simulink model "boundedModel"  (R2019a)
settings: Solver=FixedStepAuto  StartTime=0.0  StopTime=10  FixedStep=0.001  RelTol=1e-3
settings Model: Creator=houte  LastModifiedBy=coeng

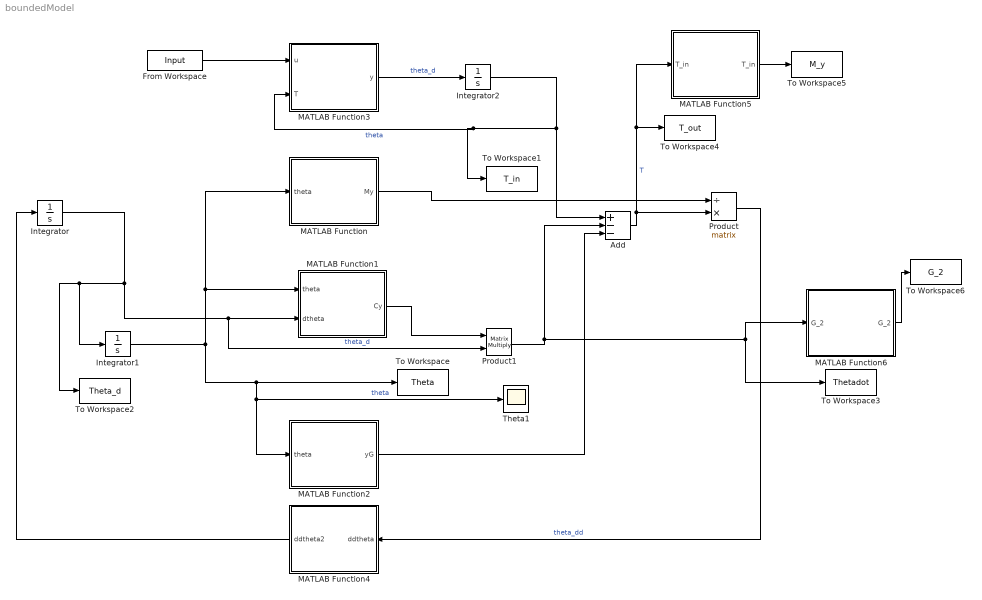
== system boundedModel ==
  Add : Sum  Inputs=+--
  From Workspace : FromWorkspace  VariableName=Input  SampleTime=0
  Integrator : Integrator  InitialCondition=[0; 0]
  Integrator1 : Integrator  InitialCondition=[0;pi]
  Integrator2 : Integrator  InitialCondition=[0;0]
  MATLAB Function : MATLAB Function  TreatAsAtomicUnit=on
  MATLAB Function1 : MATLAB Function  TreatAsAtomicUnit=on
  MATLAB Function2 : MATLAB Function  TreatAsAtomicUnit=on
  MATLAB Function3 : MATLAB Function  TreatAsAtomicUnit=on
  MATLAB Function4 : MATLAB Function  TreatAsAtomicUnit=on
  MATLAB Function5 : MATLAB Function  TreatAsAtomicUnit=on
  MATLAB Function6 : MATLAB Function  TreatAsAtomicUnit=on
  Product : Product  Inputs=/*  Multiplication=Matrix(*)
  Product1 : Product  Multiplication=Matrix(*)
  Theta1 : Scope
  To Workspace : ToWorkspace  VariableName=Theta  SaveFormat=Timeseries  SampleTime=-1
  To Workspace1 : ToWorkspace  VariableName=T_in  SaveFormat=Timeseries  SampleTime=-1
  To Workspace2 : ToWorkspace  VariableName=Theta_d  SaveFormat=Timeseries  SampleTime=-1
  To Workspace3 : ToWorkspace  VariableName=Thetadot  SaveFormat=Timeseries  SampleTime=-1
  To Workspace4 : ToWorkspace  VariableName=T_out  SaveFormat=Timeseries  SampleTime=-1
  To Workspace5 : ToWorkspace  VariableName=M_y  SaveFormat=Timeseries  SampleTime=-1
  To Workspace6 : ToWorkspace  VariableName=G_2  SaveFormat=Timeseries  SampleTime=-1
  wires:
  Integrator/1 -> To Workspace2/1, Integrator1/1, Product1/2, MATLAB Function1/2(dtheta)  "theta_d"
  Integrator1/1 -> MATLAB Function/1(theta), MATLAB Function1/1(theta), MATLAB Function2/1(theta), Theta1/1, To Workspace/1  "theta"
  Add/1 -> MATLAB Function5/1("T_in "), To Workspace4/1, Product/2  "T"
  MATLAB Function1/1(Cy) -> Product1/1
  MATLAB Function2/1(yG) -> Add/3
  MATLAB Function/1(My) -> Product/1
  Product/1 -> MATLAB Function4/1(ddtheta)  "theta_dd"
  MATLAB Function3/1(y) -> Integrator2/1  "theta_d"
  Product1/1 -> Add/2, MATLAB Function6/1("G_2 "), To Workspace3/1
  From Workspace/1 -> MATLAB Function3/1(u)
  MATLAB Function4/1(ddtheta2) -> Integrator/1
  MATLAB Function5/1(T_in) -> To Workspace5/1
  MATLAB Function6/1(G_2) -> To Workspace6/1
  Integrator2/1 -> MATLAB Function3/2(T), To Workspace1/1, Add/1  "theta"

== matlab function boundedModel/MATLAB Function1 ==
  data: theta input; Cy output; dtheta input; Parameters parameter
function Cy = C(theta, dtheta, Parameters)
    theta1 = theta(1);
    theta2 = theta(2);
    dtheta1 = dtheta(1);
    dtheta2 = dtheta(2);

Cy = [Parameters.b1 - Parameters.P3*dtheta2*sin(theta2), -Parameters.P3*(dtheta1+dtheta2)*sin(theta2);
    Parameters.P3*dtheta1*sin(theta2), Parameters.b2];

== matlab function boundedModel/MATLAB Function ==
  data: theta input; My output; Parameters parameter
function My = M(theta, Parameters)
theta1 = theta(1);
theta2 = theta(2);

My = [Parameters.P1 + Parameters.P2 + 2*Parameters.P3*cos(theta2), Parameters.P2 + Parameters.P3 * cos(theta2);
     Parameters.P2 + Parameters.P3*cos(theta2), Parameters.P2];
 detY = det(My);

== matlab function boundedModel/MATLAB Function2 ==
  data: theta input; yG output; Parameters parameter
function yG = G(theta, Parameters)
    theta1 = theta(1);
    theta2 = theta(2);

yG = [-Parameters.g1*sin(theta1) - Parameters.g2*sin(theta1+theta2);
     -Parameters.g2*sin(theta1+theta2)];

== matlab function boundedModel/MATLAB Function3 ==
  data: u input; y output; Parameters parameter; T input
function y = T(u, Parameters, T)
    T_old = T;
    % T = km*u - Te*dTe;
    %dTe = (km*u-T)/Te
    dTe = (Parameters.km*u-T(1))/Parameters.Te;
    Tn = u/Parameters.km/1000;
y = [dTe; 0];

== matlab function boundedModel/MATLAB Function4 ==
  data: ddtheta input; ddtheta2 output; Parameters parameter
function ddtheta2 = M(ddtheta, Parameters)
ddtheta2 = [ddtheta(1); 0];

== matlab function boundedModel/MATLAB Function5 ==
  data: T_in input; T_in output; Parameters parameter
function T_in = M(T_in, Parameters)

T_in = T_in;

== matlab function boundedModel/MATLAB Function6 ==
  data: G_2 input; G_2 output; Parameters parameter
function G_2 = M(G_2, Parameters)

G_2 = G_2;
